simulink model "Q1_a"  (R2020b)
settings: Solver=VariableStepAuto  StartTime=0.0  StopTime=60.0  RelTol=1e-3
settings Model: Creator=aloks  LastModifiedBy=aloks

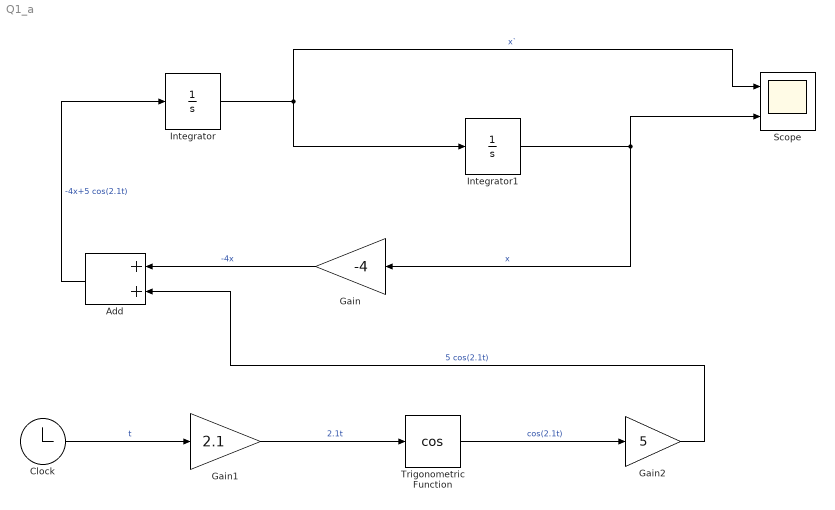
== system Q1_a ==
  Add : Sum
  Clock : Clock
  Gain : Gain  Gain=-4
  Gain1 : Gain  Gain=2.1
  Gain2 : Gain  Gain=5
  Integrator : Integrator  InitialCondition=1
  Integrator1 : Integrator  InitialCondition=2
  Scope : Scope  NumInputPorts=2
  Trigonometric Function : Trigonometry  Operator=cos
  wires:
  Integrator/1 -> Scope/1, Integrator1/1  "x`"
  Integrator1/1 -> Scope/2, Gain/1  "x"
  Clock/1 -> Gain1/1  "t"
  Gain1/1 -> Trigonometric Function/1  "2.1t"
  Trigonometric Function/1 -> Gain2/1  "cos(2.1t)"
  Gain/1 -> Add/1  "-4x"
  Add/1 -> Integrator/1  "-4x+5 cos(2.1t)"
  Gain2/1 -> Add/2  "5 cos(2.1t)"
